simulink model "friction_model"  (R2023a)
settings: Solver=VariableStepAuto  StartTime=0.0  StopTime=10.0  RelTol=1e-3
values from neighbouring files (symbols this model uses):
  b = K_t / average_Kt_b    [current_velocity_model.m]    (also in current_velocity_tf.m = -1 * m * log10(LARGE_FREQUENCY) + large_w_M; params_from_chirp.m = -1 * m * log10(LARGE_FREQUENCY) + large_w_M)
  J = 0.5 * mass * radius * radius    (= 0.000549334964416)    [calculateJ.m]    (also in current_velocity_model.m = average_J_b * b; damping_from_steps.m)
  K_t = 0.1    [current_velocity_model.m]    (also in damping_from_steps.m; friction_from_steps.m)
undefined symbols (not defined in the file or in its folder): F_c
settings Model: Creator=yunzh  LastModifiedBy=yunzh

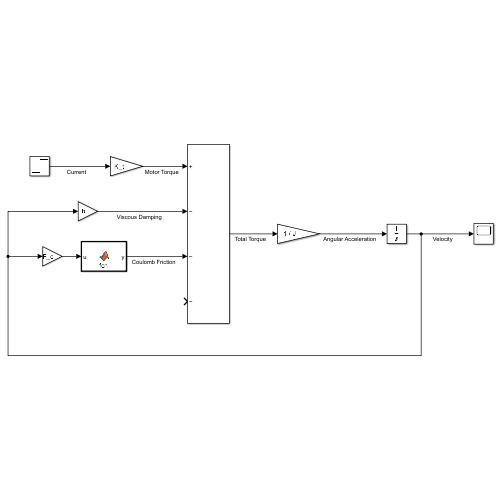
[thumbnail: Simulink's stored preview of the top-level diagram]
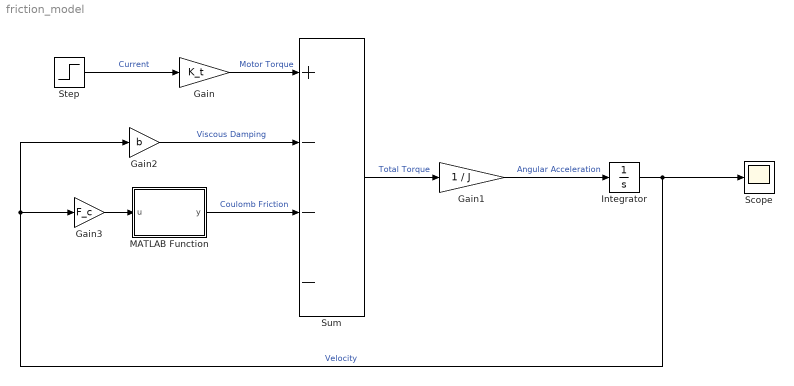
== system friction_model ==
  Gain : Gain  Gain=K_t
  Gain1 : Gain  Gain=1 / J
  Gain2 : Gain  Gain=b
  Gain3 : Gain  Gain=F_c
  Integrator : Integrator
  MATLAB Function : MATLAB Function  TreatAsAtomicUnit=on
  Scope : Scope
  Step : Step  SampleTime=0
  Sum : Sum  Inputs=+---
  wires:
  Gain/1 -> Sum/1  "Motor Torque"
  Step/1 -> Gain/1  "Current"
  Sum/1 -> Gain1/1  "Total Torque"
  Gain2/1 -> Sum/2  "Viscous Damping"
  Gain1/1 -> Integrator/1  "Angular Acceleration"
  Integrator/1 -> Scope/1, Gain2/1, Gain3/1  "Velocity"
  MATLAB Function/1(y) -> Sum/3  "Coulomb Friction"
  Gain3/1 -> MATLAB Function/1(u)

== matlab function friction_model/MATLAB Function ==
  data: u input; y output
function y = fcn(u)
    EPSILON = 0.005;

    if u < EPSILON
        y = 0;
        return;
    end

    y = sign(u);
